simulink model "kadai12"  (R2021b)
settings: Solver=VariableStepAuto  StartTime=0.0  StopTime=2.5  RelTol=1e-3
settings Model: Creator=is221042  LastModifiedBy=tomotomo

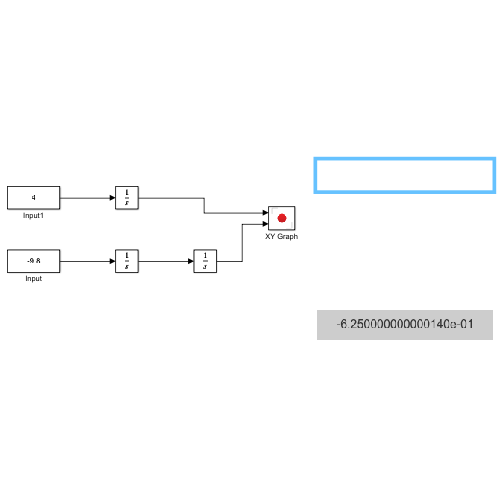
[thumbnail: Simulink's stored preview of the top-level diagram]
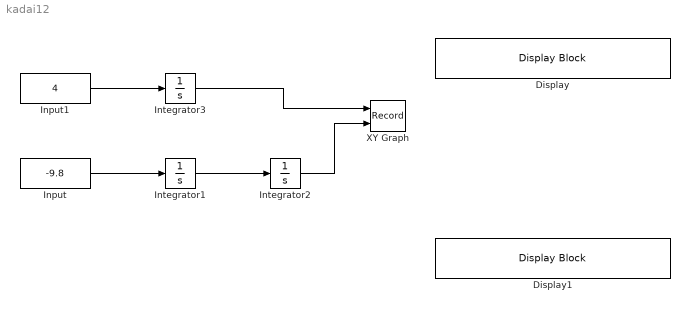
== system kadai12 ==
  Display : DisplayBlock  LabelPosition=Hide  Format=longE  Transparency=1
  Display1 : DisplayBlock  LabelPosition=Hide  Format=longE  Transparency=1
  Input : Constant  Value=-9.8
  Input1 : Constant  Value=4
  Integrator1 : Integrator  InitialCondition=12
  Integrator2 : Integrator
  Integrator3 : Integrator
  XY Graph : Record  FileSettingsInternal="{\"entries\":[{\"content\":{\"excelSettings\":{\"content\":{},\"type\":\"Streamout.ExcelSettings\"}},\"type\":\"Streamout.FileSettingStorage\",\"uuid\":\"c32a3880-fb3b-4032-960b-f268b8ea9eb9\"}],\"packageUris\":[\"http://schema.mathworks.com/mf0/streamout_blocks/R2020a\"],\"version\":\"1.0\"}"  Layout=[1 1]  SignalsInternal="{\"entries\":[{\"content\":{\"signals\":[{\"content\":{\"blockPath\":[\"kadai12/XY Graph\"],\"channel\":[],\"dimensions\":[1],\"domain\":\"kadai12/XY Graph\",\"lineColor\":\"#a2142f\",\"plots\":[1],\"port\":1,\"sid\":[\"\"],\"signalID\":5449,\"signalName\":\"Integrator3\"},\"type\":\"RecordBlkView.Signal\",\"uuid\":\"f0cf2c37-c71e-40c0-af24-aecddc7be472\"},{\"content\":{\"blockPath\":[\"kadai12/XY Graph\"],\"channel\":[],\"dimensions\":[1],\"domain\":\"kadai12/XY Graph\",\"lineColor\":\"#139fff\",\"plots\":[1],\"port\":2,\"sid\":[\"\"],\"signalID\":5453,\"signalName\":\"Integrator2\"},\"type\":\"RecordBlkView.Signal\",\"uuid\":\"b5120ea1-1dd9-4af5-beef-235bb32d9734\"}]},\"type\":\"RecordBlkView.InputSignals\",\"uuid\":\"91b66e53-bb6a-40af-b4e4-bee9483a2132\"}],\"packageUris\":[\"http://schema.mathworks.com/mf0/streamout_blocks/R2020a\"],\"version\":\"1.0\"}"  VisualizationBindings="{\"xyplotplugin\":{\"info\":[{\"series\":[{\"bindingParametersList\":[{\"parameter\":\"X-Axis\",\"signalID\":5449,\"signalName\":\"Integrator3\"},{\"parameter\":\"Y-Axis\",\"signalID\":5453,\"signalName\":\"Integrator2\"}],\"seriesID\":5268}],\"subplotID\":1}]}}"  CompatibilityTag=XY
  wires:
  Input/1 -> Integrator1/1
  Integrator3/1 -> XY Graph/1
  Integrator2/1 -> XY Graph/2
  Input1/1 -> Integrator3/1
  Integrator1/1 -> Integrator2/1
